simulink library "powerlib_models"  (Simulink 6.0)
settings: Solver=ode45  SolverMode=SingleTasking  StartTime=0.0  StopTime=10.0  RelTol=1e-3
values from neighbouring files (symbols this model uses):
  Ts = get(handles.edit1,'string')    [powergui.m]
undefined symbols (not defined in the file or in its folder): A, a0, a1, a2, a3, a4, a5, Ac, Amplitude, Amplitudes, B, BaseCurrent, BaseFlux, Bc, C, Capacitance, Cc, Columns, ConnectionType, Cs, ctrl, current, Current, damp, Dc, Dd, DiscIntNeverNeededParam, dref, dwo, exc, excAxis, F, Flux, fnom, Frequency, FreqVps, Gain1, gate, GH, GHd, GI, GId, GL, GLd, H, HarmonicGeneration, HT, hyd, I1_init, ib, ib2, Id1o, Inductance, InitialFlux, InitialSlope, io, Iq1o, isfinite, j, J ... (+138)
libraries: powerlib_models x32, powerlib_extras x4
(part 5 of 11)

== system powerlib_models/Phasors/SM_mechanics ==
  note: This subsystem models the mechanical part of the machine.
  Te : Inport  Port=1  PortDimensions=1  LatchInput=off
  Pm : Inport  Port=2  LatchInput=off
  1_(2H) : Gain  Gain=1/(2*H)  SaturateOnIntegerOverflow=on
  1_Pb : Gain  Gain=1/Pb  SaturateOnIntegerOverflow=on
  Clock : Clock
      settings: Decimation=10
  F1 : Gain  Orientation=left  Gain=F  SaturateOnIntegerOverflow=on
  Integrator : Integrator  InitialCondition=dwo
  Integrator1 : Integrator  InitialCondition=tho
  Integrator2 : Integrator  InitialCondition=tho
  Mux1 : Mux  Inputs=2
  Mux2 : Mux  Inputs=6
  Product : Product  SaturateOnIntegerOverflow=on  InputSameDT=on
  Sum : Sum  SaturateOnIntegerOverflow=on  InputSameDT=on
  Sum2 : Sum  Inputs=+--  SaturateOnIntegerOverflow=on  InputSameDT=on
  Sum3 : Sum  SaturateOnIntegerOverflow=on  InputSameDT=on
  div : Fcn  Expr=u[2]/u[1]
      mask Display: disp('/')
  nom. speed : Constant
  theta : Gain  Gain=180/pi  SaturateOnIntegerOverflow=on
  units : Gain  Gain=Nb  SaturateOnIntegerOverflow=on
  units1 : Gain  Gain=Pb  SaturateOnIntegerOverflow=on
  units2 : Gain  Gain=Pb/Nb  SaturateOnIntegerOverflow=on
  web1 : Gain  Gain=web_psb  SaturateOnIntegerOverflow=on
  web2 : Gain  Gain=web_psb  SaturateOnIntegerOverflow=on
  web3 : Gain  Gain=web_psb  SaturateOnIntegerOverflow=on
  misc : Outport  InitialOutput=0
  thetae : Outport  Port=2  InitialOutput=0
  we : Outport  Port=3  InitialOutput=0
  wires:
  Sum3/1 -> thetae/1
  Mux2/1 -> misc/1
  Sum/1 -> F1/1, Product/1, web3/1, units/1, Mux1/1, we/1  "n"
  Sum2/1 -> 1_(2H)/1
  F1/1 -> Sum2/3
  1_Pb/1 -> Mux1/2
  Pm/1 -> 1_Pb/1
  Mux1/1 -> div/1
  Te/1 -> Product/2, Sum2/2, units2/1  "Te"
  div/1 -> Sum2/1
  1_(2H)/1 -> Integrator/1
  nom. speed/1 -> Sum/1
  Product/1 -> units1/1  "Pe"
  Integrator/1 -> Sum/2, web1/1, Mux2/4  "dw"
  web1/1 -> Integrator2/1
  Clock/1 -> web2/1
  web2/1 -> Sum3/2
  Integrator2/1 -> Sum3/1, Mux2/1  "d_theta (rad)"
  Integrator1/1 -> theta/1  "d_theta (rad)"
  web3/1 -> Integrator1/1
  theta/1 -> Mux2/5  "theta"
  units/1 -> Mux2/2
  units1/1 -> Mux2/3
  units2/1 -> Mux2/6

== system powerlib_models/Phasors/SSM_mechanics ==
  Pm : Inport  Port=1  LatchInput=off
  Pe : Inport  Port=2  LatchInput=off
  1_(2*H) : Gain  Gain=1/(2*H)  SaturateOnIntegerOverflow=on
  1_Pb : Gain  Gain=1/Pb  SaturateOnIntegerOverflow=on
  Gain : Gain  Orientation=left  Gain=Kd  SaturateOnIntegerOverflow=on
  Integrator : Integrator  InitialCondition=dwo
  Integrator1 : Integrator  InitialCondition=tho
  Mux1 : Mux  Inputs=2
  Sum : Sum  SaturateOnIntegerOverflow=on  InputSameDT=on
  Sum1 : Sum  Inputs=+-  SaturateOnIntegerOverflow=on  InputSameDT=on
  Sum2 : Sum  Inputs=-+  SaturateOnIntegerOverflow=on  InputSameDT=on
  div : Fcn  Expr=u[2]/u[1]
      mask Display: disp('division')
  nom. speed : Constant
  web : Gain  Gain=web  SaturateOnIntegerOverflow=on
  theta_e : Outport  InitialOutput=0
  wm : Outport  Port=2  InitialOutput=0
  wires:
  nom. speed/1 -> Sum/1
  Integrator/1 -> Gain/1, Sum/2
  Sum1/1 -> 1_(2*H)/1
  Gain/1 -> Sum1/2
  div/1 -> Sum1/1
  1_(2*H)/1 -> Integrator/1
  Sum/1 -> web/1, wm/1, Mux1/1
  Sum2/1 -> Mux1/2
  Pe/1 -> Sum2/1
  Mux1/1 -> div/1
  Integrator1/1 -> theta_e/1
  web/1 -> Integrator1/1
  1_Pb/1 -> Sum2/2
  Pm/1 -> 1_Pb/1

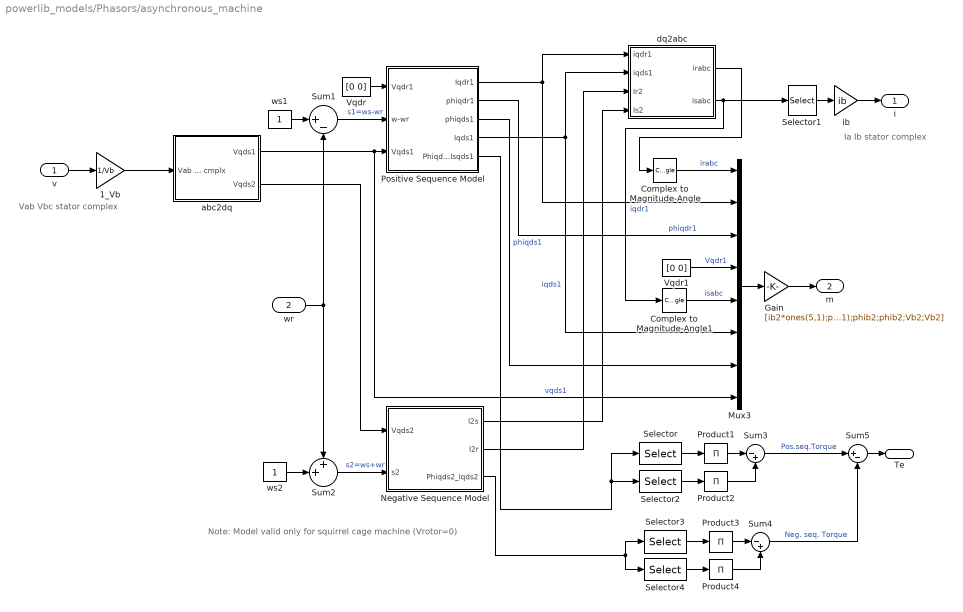
== system powerlib_models/Phasors/asynchronous_machine ==
  note: Note: Model valid only for squirrel cage machine (Vrotor=0)
  note: Ia Ib stator
      | complex
  note: Vab Vbc stator
      | complex
  v : Inport  Port=1  LatchInput=off
  wr : Inport  Port=2  LatchInput=off
  1_Vb : Gain  Gain=1/Vb  SaturateOnIntegerOverflow=on
  Complex to Magnitude-Angle : ComplexToMagnitudeAngle  Output=Magnitude
  Complex to Magnitude-Angle1 : ComplexToMagnitudeAngle  Output=Magnitude
  Gain : Gain  Gain=[ib2*ones(5,1);phib2;phib2;Vb2;Vb2;ib2*ones(5,1);phib2;phib2;Vb2;Vb2]  SaturateOnIntegerOverflow=on
  Mux3 : Mux  Inputs=[3,2,2,2,3,2,2,2]
  Negative Sequence Model : Subsystem
  Positive Sequence Model : Subsystem
  Product{1..4} (4 alike) : Product  Inputs=1  SaturateOnIntegerOverflow=on  InputSameDT=on
  Selector : Selector  Elements=[1 4]  InputPortWidth=4
  Selector1 : Selector  Elements=[1 2]  InputPortWidth=3
  Selector2 : Selector  Elements=[2 3]  InputPortWidth=4
  Selector3 : Selector  Elements=[1 4]  InputPortWidth=4
  Selector4 : Selector  Elements=[2 3]  InputPortWidth=4
  Sum1 : Sum  Inputs=|+-  SaturateOnIntegerOverflow=on  InputSameDT=on
  Sum2 : Sum  Inputs=++|  SaturateOnIntegerOverflow=on  InputSameDT=on
  Sum3 : Sum  Inputs=|-+  SaturateOnIntegerOverflow=on  InputSameDT=on
  Sum4 : Sum  Inputs=|-+  SaturateOnIntegerOverflow=on  InputSameDT=on
  Sum5 : Sum  Inputs=|+-  SaturateOnIntegerOverflow=on  InputSameDT=on
  Vqdr : Constant  Value=[0 0]
  Vqdr1 : Constant  Value=[0 0]
  abc2dq : Subsystem
  dq2abc : Subsystem
  ib : Gain  Gain=ib  SaturateOnIntegerOverflow=on
  ws1 : Constant
  ws2 : Constant
  i : Outport
  m : Outport  Port=2
  Te : Outport  Port=3
  wires:
  Negative Sequence Model/2(I2r) -> dq2abc/3(Ir2)
  Negative Sequence Model/1(I2s) -> dq2abc/4(Is2)
  Positive Sequence Model/3(phiqds1) -> Mux3/7  "phiqds1"
  Positive Sequence Model/2(phiqdr1) -> Mux3/3  "phiqdr1"
  abc2dq/2(Vqds2) -> Negative Sequence Model/1(Vqds2)
  Sum2/1 -> Negative Sequence Model/2(s2)  "s2=ws+wr"
  ib/1 -> i/1
  Mux3/1 -> Gain/1
  Gain/1 -> m/1
  dq2abc/2(isabc) -> Complex to Magnitude-Angle1/1, Selector1/1
  dq2abc/1(irabc) -> Complex to Magnitude-Angle/1
  Positive Sequence Model/1(Iqdr1) -> Mux3/2, dq2abc/1(iqdr1)  "iqdr1"
  abc2dq/1(Vqds1) -> Positive Sequence Model/3(Vqds1), Mux3/8  "vqds1"
  Positive Sequence Model/4(Iqds1) -> dq2abc/2(iqds1), Mux3/6  "iqds1"
  Vqdr/1 -> Positive Sequence Model/1(Vqdr1)
  1_Vb/1 -> abc2dq/1(Vab Vbc cmplx)
  v/1 -> 1_Vb/1
  Selector1/1 -> ib/1
  Complex to Magnitude-Angle/1 -> Mux3/1  "irabc"
  Complex to Magnitude-Angle1/1 -> Mux3/5  "isabc"
  ws1/1 -> Sum1/1
  Sum1/1 -> Positive Sequence Model/2(w-wr)  "s1=ws-wr"
  Vqdr1/1 -> Mux3/4  "Vqdr1"
  ws2/1 -> Sum2/2
  wr/1 -> Sum2/1, Sum1/2
  Positive Sequence Model/5(Phiqds1_Isqds1) -> Selector2/1, Selector/1
  Negative Sequence Model/3(Phiqds2_Iqds2) -> Selector3/1, Selector4/1
  Sum4/1 -> Sum5/2  "Neg. seq. Torque"
  Sum3/1 -> Sum5/1  "Pos.seq.Torque"
  Product3/1 -> Sum4/1
  Product4/1 -> Sum4/2
  Selector4/1 -> Product4/1
  Selector3/1 -> Product3/1
  Product1/1 -> Sum3/1
  Product2/1 -> Sum3/2
  Selector2/1 -> Product2/1
  Selector/1 -> Product1/1
  Sum5/1 -> Te/1

== system powerlib_models/Phasors/breaker ==
  "v " : Inport  Port=1  LatchInput=off
  g : Inport  Port=2  LatchInput=off
  Constant : Constant  Value=complex(zeros(Nsw,1),zeros(Nsw,1))
  Terminator : Terminator
  i : Outport  InitialOutput=0
  Status : Outport  Port=2  InitialOutput=0
  wires:
  Constant/1 -> i/1
  g/1 -> Status/1
  "v "/1 -> Terminator/1  "Vak"

== system powerlib_models/Phasors/distributed_param_line ==
  v : Inport  Port=1  LatchInput=off
  Constant : Constant  Value=complex(zeros(1,2*nphase),zeros(1,2*nphase))
  Terminator : Terminator
  i : Outport  InitialOutput=0
  wires:
  v/1 -> Terminator/1
  Constant/1 -> i/1

== system powerlib_models/Phasors/ideal_switch ==
  v : Inport  Port=1  LatchInput=off
  g : Inport  Port=2  LatchInput=off
  1/Rsw : Gain  Gain=1./Rsw  SaturateOnIntegerOverflow=on
  1/Rsw1 : Gain  Gain=0  SaturateOnIntegerOverflow=on
  Constant : Constant  Value=complex(zeros(Nsw,1),zeros(Nsw,1))
  Mux : Mux  Inputs=2
  Switch : Switch  Threshold=0.5  InputSameDT=on
  i : Outport  InitialOutput=0
  Status : Outport  Port=2  InitialOutput=0
  m : Outport  Port=3  InitialOutput=0
  wires:
  1/Rsw1/1 -> Switch/3
  Switch/1 -> Mux/1
  1/Rsw/1 -> Switch/1  "Iak"
  v/1 -> Mux/2, 1/Rsw/1, 1/Rsw1/1  "Vak"
  Mux/1 -> m/1  "measurement signals"
  g/1 -> Status/1, Switch/2
  Constant/1 -> i/1

== system powerlib_models/Phasors/simplified_sync_mach ==
  note: ia ib complex
  note: Vab Vbc
      | complex
  v : Inport  Port=1  LatchInput=off
  e : Inport  Port=2  LatchInput=off
  theta_e : Inport  Orientation=left  Port=3  LatchInput=off
  wm : Inport  Port=4  LatchInput=off
  1_Vb : Gain  Gain=1/Vb  SaturateOnIntegerOverflow=on
  Complex to Magnitude-Angle : ComplexToMagnitudeAngle  Output=Magnitude
  Complex to Magnitude-Angle1 : ComplexToMagnitudeAngle  Output=Magnitude
  Constant4 : Constant  Orientation=left  Value=web
  Filter_T=1ms : StateSpace  A=-1e3*eye(3)  B=1e3*eye(3)  C=eye(3)  D=zeros(3)
  "Idq1 Idq2 Pe " : Subsystem
  Integrator : Integrator  Orientation=left
  LL2LN : Subsystem
  Mux1 : Mux  Inputs=3
  Phasors Ia Ib : Subsystem
  Subsystem : Subsystem
  Sum6 : Sum  Orientation=left  Inputs=+-  SaturateOnIntegerOverflow=on  InputSameDT=on
  ib1 : Gain  Gain=ib  SaturateOnIntegerOverflow=on
  i : Outport  InitialOutput=0
  m : Outport  Port=2  InitialOutput=0
  Pe : Outport  Port=3  InitialOutput=0
  wires:
  Mux1/1 -> Subsystem/3(e)
  Complex to Magnitude-Angle1/1 -> Filter_T=1ms/1
  LL2LN/1(Vabc_n) -> Complex to Magnitude-Angle1/1  "Line-to-neutral voltages"
  Complex to Magnitude-Angle/1 -> Subsystem/1(i)
  Phasors Ia Ib/1(Iabc cmplx) -> Complex to Magnitude-Angle/1
  "Idq1 Idq2 Pe "/1(Pe) -> Subsystem/6(Pe), Pe/1  "Pe"
  Sum6/1 -> Subsystem/4(theta), "Idq1 Idq2 Pe "/3(delta)  "theta"
  Integrator/1 -> Sum6/2
  Constant4/1 -> Integrator/1
  ib1/1 -> i/1
  Phasors Ia Ib/2(Iab cmplx) -> ib1/1
  e/1 -> Mux1/3, Mux1/1, Mux1/2, "Idq1 Idq2 Pe "/2(e)  "Internal volltage  magnitudes"
  1_Vb/1 -> LL2LN/1(Vab_bc), "Idq1 Idq2 Pe "/1(Vab Vbc cmplx)
  v/1 -> 1_Vb/1
  Subsystem/1(*) -> m/1
  "Idq1 Idq2 Pe "/2(Idq1) -> Phasors Ia Ib/1(Idq1)
  "Idq1 Idq2 Pe "/3(Idq2) -> Phasors Ia Ib/2(Idq2)
  Filter_T=1ms/1 -> Subsystem/2(v)
  theta_e/1 -> Sum6/1
  wm/1 -> Subsystem/5(wm)

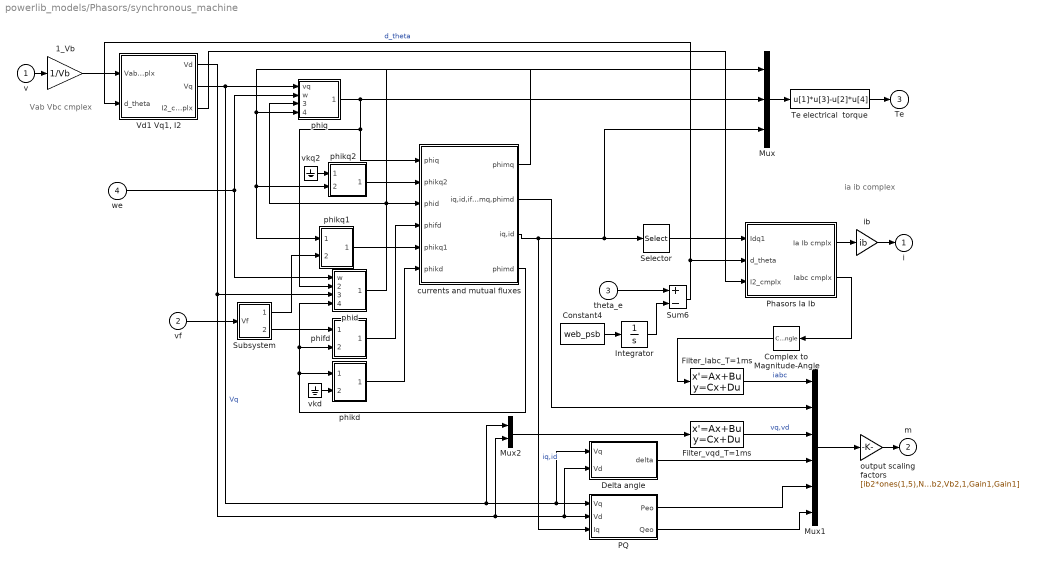
== system powerlib_models/Phasors/synchronous_machine ==
  note: Vab Vbc cmplex
  note: ia ib complex
  v : Inport  Port=1  LatchInput=off
  vf : Inport  Port=2  LatchInput=off
  theta_e : Inport  Port=3  LatchInput=off
  we : Inport  Port=4  LatchInput=off
  1_Vb : Gain  Gain=1/Vb  SaturateOnIntegerOverflow=on
  Complex to Magnitude-Angle : ComplexToMagnitudeAngle  Orientation=left  Output=Magnitude
  Constant4 : Constant  Value=web_psb
  Delta angle : Subsystem
  Filter_Iabc_T=1ms : StateSpace  A=-1e3*eye(3)  B=1e3*eye(3)  C=eye(3)  D=zeros(3)
  Filter_vqd_T=1ms : StateSpace  A=-1e3*eye(2)  B=1e3*eye(2)  C=eye(2)  D=zeros(2)  X0=[phido -phiqo]
  Integrator : Integrator
  Mux : Mux  Inputs=[ 1 1 2 ]
  Mux1 : Mux  Inputs="[ 3 8 2  1 1 1]"
  Mux2 : Mux  Inputs=2
  PQ : Subsystem
  Phasors Ia Ib : Subsystem
  Selector : Selector  Elements=[2 1]  InputPortWidth=2
  Subsystem : Subsystem
  Sum6 : Sum  Inputs=+-  SaturateOnIntegerOverflow=on  InputSameDT=on
  Te electrical  torque : Fcn  Expr=u[1]*u[3]-u[2]*u[4]
  "Vd1 Vq1, I2 " : Subsystem
  currents and mutual fluxes : Subsystem
  ib : Gain  Gain=ib  SaturateOnIntegerOverflow=on
  output scaling factors : Gain  Gain=[ib2*ones(1,5),N2,ib2,ib2,ib2,phib,phib,Vb2,Vb2,1,Gain1,Gain1]
  phid : Subsystem
      mask Display: disp('phid')
  phifd : Subsystem
      mask Display: disp('phifd')
  phikd : Subsystem
      mask Display: disp('phikd')
  phikq1 : Subsystem
      mask Display: disp('phikq1')
  phikq2 : Subsystem
      mask Display: disp('phikq2')
  phiq : Subsystem
      mask Display: disp('phiq')
  vkd : Ground
  vkq2 : Ground
  i : Outport  InitialOutput=0
  m : Outport  Port=2  InitialOutput=0
  Te : Outport  Port=3  InitialOutput=0
  wires:
  PQ/2(Qeo) -> Mux1/6
  PQ/1(Peo) -> Mux1/5
  Delta angle/1(delta) -> Mux1/4
  Complex to Magnitude-Angle/1 -> Filter_Iabc_T=1ms/1
  Phasors Ia Ib/2(Iabc cmplx) -> Complex to Magnitude-Angle/1
  ib/1 -> i/1
  Phasors Ia Ib/1(Ia Ib cmplx) -> ib/1
  currents and mutual fluxes/1(phimq) -> phiq/4(phimq), phikq1/1(phimq), phikq2/2(phimq)
  currents and mutual fluxes/4(phimd) -> phid/4(phimd), phifd/2(phimd), phikd/1(phimd)
  phiq/1(phiq) -> currents and mutual fluxes/1(phiq), phid/2(phiq), Mux/2
  "Vd1 Vq1, I2 "/1(Vd) -> phid/3(vd), PQ/2(Vd), Delta angle/2(Vd), Mux2/2
  "Vd1 Vq1, I2 "/2(Vq) -> phiq/1(vq), PQ/1(Vq), Delta angle/1(Vq), Mux2/1  "Vq"
  phid/1(phid) -> phiq/3(phid), currents and mutual fluxes/3(phid), Mux/1
  Selector/1 -> Phasors Ia Ib/1(Idq1)
  Mux2/1 -> Filter_vqd_T=1ms/1
  "Vd1 Vq1, I2 "/3(I2_cmplx) -> Phasors Ia Ib/3(I2_cmplx)
  Integrator/1 -> Sum6/2
  Constant4/1 -> Integrator/1
  Sum6/1 -> Phasors Ia Ib/2(d_theta), "Vd1 Vq1, I2 "/2(d_theta)  "d_theta"
  phikq2/1(phikq2) -> currents and mutual fluxes/2(phikq2)
  phikq1/1(phikq1) -> currents and mutual fluxes/5(phikq1)
  phifd/1(phifd) -> currents and mutual fluxes/4(phifd)
  phikd/1(phikd) -> currents and mutual fluxes/6(phikd)
  output scaling factors/1 -> m/1
  Mux1/1 -> output scaling factors/1
  currents and mutual fluxes/3(iq,id) -> PQ/3(Iq), Selector/1, Mux/3  "iq,id"
  currents and mutual fluxes/2("iq,id,ifd, ikq1,ikq2,ikd, phimq,phimd") -> Mux1/2
  v/1 -> 1_Vb/1
  1_Vb/1 -> "Vd1 Vq1, I2 "/1(Vab Vbc cmplx)
  Subsystem/2(Vfd) -> phifd/1(vfd)
  Subsystem/1(Vkq1) -> phikq1/2(vkq1)
  vkd/1 -> phikd/2(vkd)
  vkq2/1 -> phikq2/1(vkq2)
  vf/1 -> Subsystem/1(Vf)
  Filter_Iabc_T=1ms/1 -> Mux1/1  "iabc"
  Filter_vqd_T=1ms/1 -> Mux1/3  "vq,vd"
  theta_e/1 -> Sum6/1
  we/1 -> phid/1(w), phiq/2(w)
  Mux/1 -> Te electrical  torque/1
  Te electrical  torque/1 -> Te/1

== system powerlib_models/Sources/ThreePhaseSource ==
  Mux : Mux  Inputs=3
  Sine Wave A : Sin  Amplitude=Amplitude  Frequency=2*pi*Frequency  Phase=Phase*pi/180  SampleTime=Ts
  Sine Wave B : Sin  Amplitude=Amplitude  Frequency=2*pi*Frequency  Phase=(Phase-120)*pi/180  SampleTime=Ts
  Sine Wave C : Sin  Amplitude=Amplitude  Frequency=2*pi*Frequency  Phase=(Phase+120)*pi/180  SampleTime=Ts
  Out1 : Outport
  wires:
  Sine Wave B/1 -> Mux/2
  Sine Wave A/1 -> Mux/1
  Sine Wave C/1 -> Mux/3
  Mux/1 -> Out1/1

== system powerlib_models/Sources/ThreePhaseSource_Cmplx ==
  Constant : Constant  Value=complex(Amplitude*cos(Phase*pi/180),Amplitude*sin(Phase*pi/180))
  Constant1 : Constant  Value=complex(Amplitude*cos((Phase-120)*pi/180),Amplitude*sin((Phase-120)*pi/180))
  Constant2 : Constant  Value=complex(Amplitude*cos((Phase+120)*pi/180),Amplitude*sin((Phase+120)*pi/180))
  Mux : Mux  Inputs=3
  Out1 : Outport
  wires:
  Constant1/1 -> Mux/2
  Constant/1 -> Mux/1
  Constant2/1 -> Mux/3
  Mux/1 -> Out1/1

== system powerlib_models/Switch Current Source/IGBT ==
  v : Inport  Port=1  LatchInput=off
  g : Inport  Port=2  LatchInput=off
  Conduction Logic : Subsystem
  IC : InitialCondition  Value=IC
  Integrator : Integrator  ExternalReset=rising  InitialConditionSource=external  ShowStatePort=on
  L_device : Gain  Gain=1./Lon  SaturateOnIntegerOverflow=on
  Mux : Mux  Inputs=2
  R_device : Gain  Orientation=left  Gain=Ron  SaturateOnIntegerOverflow=on
  Switch : Switch  Threshold=eps  InputSameDT=on
  Tail : Subsystem
  Vak-VT-RT*Iak2 : Sum  Inputs=-|+|-  SaturateOnIntegerOverflow=on  InputSameDT=on
  Vf : Constant  Orientation=up  Value=Vf
  Vf1 : Constant  Value=0*IC
  Vf2 : Constant  Value=0
  i : Outport  InitialOutput=0
  m : Outport  Port=2  InitialOutput=0
  wires:
  Conduction Logic/1(status) -> Tail/2(switch), Integrator/2, Switch/2
  Integrator/1 -> R_device/1, Tail/1(iak)  "IGBT current"
  IC/1 -> Integrator/3
  Integrator/State -> Conduction Logic/1(iak)  "IGBT current"
  g/1 -> Conduction Logic/3(g)  "gate signal"
  Vak-VT-RT*Iak2/1 -> L_device/1
  Tail/1(Iak) -> Mux/1, i/1  "current"
  Mux/1 -> m/1
  Vf/1 -> Vak-VT-RT*Iak2/3
  v/1 -> Vak-VT-RT*Iak2/2, Conduction Logic/2(Vak), Mux/2  "IGBT voltage"
  R_device/1 -> Vak-VT-RT*Iak2/1
  Vf1/1 -> IC/1
  Switch/1 -> Integrator/1
  L_device/1 -> Switch/1
  Vf2/1 -> Switch/3

== system powerlib_models/Switch Current Source/detailed_thyristor ==
  v : Inport  Port=1  LatchInput=off
  g : Inport  Port=2  LatchInput=off
  Conduction logic : Subsystem
  Mux : Mux  Inputs=2
  Switch-Ron-Lon : Subsystem
  i : Outport  InitialOutput=0
  m : Outport  Port=2  InitialOutput=0
  wires:
  Conduction logic/1(reset) -> Switch-Ron-Lon/2(Reset)
  Mux/1 -> m/1
  Switch-Ron-Lon/1("Iak  ") -> i/1, Mux/1, Conduction logic/1(Iak_meas.)
  v/1 -> Switch-Ron-Lon/1(Vak), Conduction logic/2(Vak), Mux/2
  g/1 -> Conduction logic/3(G)

== system powerlib_models/Switch Current Source/diode ==
  v : Inport  Port=1  LatchInput=off
  0  1 : Constant  Value=0
  Conduction logic : Subsystem
  IC : InitialCondition  Value=IC
  Integrator1 : Integrator  ExternalReset=rising  InitialConditionSource=external  LimitOutput=on  LowerSaturationLimit=0
  Lon : Gain  Gain=1./Lon  SaturateOnIntegerOverflow=on
  Mux : Mux  Inputs=2
  Ron : Gain  Orientation=left  Gain=Ron  SaturateOnIntegerOverflow=on
  Test : Switch  Threshold=0.5  InputSameDT=on
  Vak-VT-RT*Iak2 : Sum  Inputs=-|+|-  SaturateOnIntegerOverflow=on  InputSameDT=on
  Vf : Constant  Orientation=up  Value=Vf
  Vf1 : Constant  Value=0*IC
  i : Outport  InitialOutput=0
  m : Outport  Port=2  InitialOutput=0
  wires:
  Mux/1 -> m/1
  v/1 -> Mux/2, Conduction logic/2(Vak), Vak-VT-RT*Iak2/2  "Diode voltage"
  IC/1 -> Integrator1/3
  Lon/1 -> Integrator1/1
  Conduction logic/1(status) -> Integrator1/2, Test/2
  Vak-VT-RT*Iak2/1 -> Lon/1
  Integrator1/1 -> Ron/1, Test/1  "Inductor current"
  Ron/1 -> Vak-VT-RT*Iak2/1
  Vf/1 -> Vak-VT-RT*Iak2/3
  Vf1/1 -> IC/1
  0  1/1 -> Test/3  "zero current"
  Test/1 -> i/1, Mux/1, Conduction logic/1(Iak)  "Diode current"

== system powerlib_models/Switch Current Source/gto ==
  v : Inport  Port=1  LatchInput=off
  g : Inport  Port=2  LatchInput=off
  Conduction Logic : Subsystem
  IC : InitialCondition  Value=IC
  Integrator : Integrator  ExternalReset=rising  InitialConditionSource=external  ShowStatePort=on
  L_device : Gain  Gain=1./Lon  SaturateOnIntegerOverflow=on
  Mux : Mux  Inputs=2
  R_device : Gain  Orientation=left  Gain=Ron  SaturateOnIntegerOverflow=on
  Switch : Switch  Threshold=eps  InputSameDT=on
  Tail : Subsystem
  Vak-VT-RT*Iak2 : Sum  Inputs=-|+|-  SaturateOnIntegerOverflow=on  InputSameDT=on
  Vf : Constant  Orientation=up  Value=Vf
  Vf1 : Constant  Value=0*IC
  Vf2 : Constant  Value=0
  i : Outport  InitialOutput=0
  m : Outport  Port=2  InitialOutput=0
  wires:
  Conduction Logic/1(status) -> Tail/2(switch), Integrator/2, Switch/2  "switch status"
  Integrator/1 -> Tail/1(iak), R_device/1  "GTO current"
  Integrator/State -> Conduction Logic/1(iak)  "GTO current"
  g/1 -> Conduction Logic/3(g)  "gate signal"
  R_device/1 -> Vak-VT-RT*Iak2/1
  Tail/1(Iak) -> i/1, Mux/1  "GTO current"
  Mux/1 -> m/1
  v/1 -> Vak-VT-RT*Iak2/2, Mux/2, Conduction Logic/2(Vak)  "GTO voltage"
  Vf/1 -> Vak-VT-RT*Iak2/3
  Vak-VT-RT*Iak2/1 -> L_device/1
  Vf1/1 -> IC/1
  IC/1 -> Integrator/3
  Switch/1 -> Integrator/1
  L_device/1 -> Switch/1
  Vf2/1 -> Switch/3

== system powerlib_models/Switch Current Source/mosfet ==
  v : Inport  Port=1  LatchInput=off
  g : Inport  Port=2  LatchInput=off
  0  1 : Constant  Value=0
  Conduction Logic : Subsystem
  IC : InitialCondition  Value=IC
  Integrator1 : Integrator  ExternalReset=rising  InitialConditionSource=external  LowerSaturationLimit=0  ShowStatePort=on
  Lon : Gain  Gain=1./Lon  SaturateOnIntegerOverflow=on
  Mux : Mux  Inputs=2
  R_device : Gain  Orientation=left  Gain=Ron  SaturateOnIntegerOverflow=on
  R_device1 : Gain  Orientation=left  Gain=Rd  SaturateOnIntegerOverflow=on
  Sign : Signum  Orientation=left
  Test : Switch  Threshold=0.5  InputSameDT=on
  Test4 : Switch  Orientation=left  Threshold=eps  InputSameDT=on
  Vds-Ron*Ids : Sum  Inputs=-+|  SaturateOnIntegerOverflow=on  InputSameDT=on
  Vf1 : Constant  Value=0*IC
  i : Outport  InitialOutput=0
  m : Outport  Port=2  InitialOutput=0
  wires:
  Integrator1/1 -> Test/1, Sign/1, R_device/1, R_device1/1  "mosfet current"
  Test/1 -> Mux/1, i/1
  Conduction Logic/1(status) -> Integrator1/2, Test/2
  Integrator1/State -> Conduction Logic/1(Ids_meas)  "mosfet current"
  v/1 -> Mux/2, Conduction Logic/2(Vds), Vds-Ron*Ids/2  "mosfet voltage"
  Sign/1 -> Test4/2
  R_device1/1 -> Test4/3
  Lon/1 -> Integrator1/1
  Vds-Ron*Ids/1 -> Lon/1
  R_device/1 -> Test4/1
  g/1 -> Conduction Logic/3(G)  "gate signal"
  Mux/1 -> m/1
  Test4/1 -> Vds-Ron*Ids/1
  0  1/1 -> Test/3  "zero current"
  Vf1/1 -> IC/1
  IC/1 -> Integrator1/3

== system powerlib_models/Switch Current Source/thyristor ==
  v : Inport  Port=1  LatchInput=off
  g : Inport  Port=2  LatchInput=off
  0  1 : Constant  Value=0
  Conduction Logic : Subsystem
  IC : InitialCondition  Value=IC
  Integrator : Integrator  ExternalReset=rising  InitialConditionSource=external  LimitOutput=on  LowerSaturationLimit=0
  Lon : Gain  Gain=1./Lon  SaturateOnIntegerOverflow=on
  Mux : Mux  Inputs=2
  R_device : Gain  Orientation=left  Gain=Ron  SaturateOnIntegerOverflow=on
  Test : Switch  Threshold=0.5  InputSameDT=on
  Vak-VT-RT*Iak2 : Sum  Inputs=-|+|-  SaturateOnIntegerOverflow=on  InputSameDT=on
  Vf : Constant  Orientation=up  Value=Vf
  Vf1 : Constant  Value=0*IC
  i : Outport  InitialOutput=0
  m : Outport  Port=2  InitialOutput=0
  wires:
  g/1 -> Conduction Logic/3("G ")  "gate signal"
  Conduction Logic/1(Status) -> Integrator/2, Test/2
  Mux/1 -> m/1
  Lon/1 -> Integrator/1
  Integrator/1 -> R_device/1, Test/1  "Inductor current"
  v/1 -> Conduction Logic/2(Vak), Mux/2, Vak-VT-RT*Iak2/2  "thyristor voltage"
  Vak-VT-RT*Iak2/1 -> Lon/1
  IC/1 -> Integrator/3
  R_device/1 -> Vak-VT-RT*Iak2/1
  Vf/1 -> Vak-VT-RT*Iak2/3
  Vf1/1 -> IC/1
  Test/1 -> i/1, Mux/1, Conduction Logic/1("Iak ")  "Thyiristor Current"
  0  1/1 -> Test/3  "zero current"

== system powerlib_models/Continuous/3_Phase_Prog_Source/Harmonic A generation ==
  Enable : Inport  Port=1  LatchInput=off
  Clock : Clock
  Gain2 : Gain  Gain=2*pi*n_Harmo  SaturateOnIntegerOverflow=on
  Gain3 : Gain  Gain=pi/180  SaturateOnIntegerOverflow=on
  Multiport Switch : MultiPortSwitch  Inputs=3  InputSameDT=on
  Negative-sequence : Constant  Value=[0 2*pi/3 -2*pi/3]
  Phase_Harmo : Constant  Value=Phase_Harmo
  Phase_Harmo1 : Constant  Value=Mag_Harmo
  Phase_Harmo2 : Constant  Value=Seq_Harmo
  Positive-sequence : Constant  Value=[0 -2*pi/3 2*pi/3]
  Product : Product  SaturateOnIntegerOverflow=on  InputSameDT=on
  Product1 : Product  Inputs=3  SaturateOnIntegerOverflow=on  InputSameDT=on
  Sum : Sum  Inputs=+++  SaturateOnIntegerOverflow=on  InputSameDT=on
  Sum1 : Sum  SaturateOnIntegerOverflow=on  InputSameDT=on
  Trigonometric Function1 : Trigonometry
  Zero-sequence : Constant  Value=[0 0 0]
  valp_nom1 : Constant  Value=Freq_Vps
  valp_nom2 : Constant
  HarmoA : Outport
  wires:
  Gain3/1 -> Sum/2
  Phase_Harmo/1 -> Gain3/1
  Enable/1 -> Product1/1
  valp_nom2/1 -> Sum1/2
  Phase_Harmo2/1 -> Sum1/1
  Sum1/1 -> Multiport Switch/1
  Phase_Harmo1/1 -> Product1/2
  Product1/1 -> HarmoA/1
  Trigonometric Function1/1 -> Product1/3
  Product/1 -> Sum/1
  Clock/1 -> Product/1
  Gain2/1 -> Product/2
  valp_nom1/1 -> Gain2/1
  Negative-sequence/1 -> Multiport Switch/4
  Positive-sequence/1 -> Multiport Switch/3
  Zero-sequence/1 -> Multiport Switch/2
  Multiport Switch/1 -> Sum/3
  Sum/1 -> Trigonometric Function1/1

== system powerlib_models/Continuous/3_Phase_Prog_Source/Harmonic B generation ==
  Enable : Inport  Port=1  LatchInput=off
  Clock1 : Clock
  Gain2 : Gain  Gain=2*pi*n_Harmo  SaturateOnIntegerOverflow=on
  Gain3 : Gain  Gain=pi/180  SaturateOnIntegerOverflow=on
  Multiport Switch : MultiPortSwitch  Inputs=3  InputSameDT=on
  Negative-sequence : Constant  Value=[0 2*pi/3 -2*pi/3]
  Phase_Harmo : Constant  Value=Phase_Harmo
  Phase_Harmo1 : Constant  Value=Mag_Harmo
  Phase_Harmo2 : Constant  Value=Seq_Harmo
  Positive-sequence : Constant  Value=[0 -2*pi/3 2*pi/3]
  Product : Product  SaturateOnIntegerOverflow=on  InputSameDT=on
  Product1 : Product  Inputs=3  SaturateOnIntegerOverflow=on  InputSameDT=on
  Sum : Sum  Inputs=+++  SaturateOnIntegerOverflow=on  InputSameDT=on
  Sum1 : Sum  SaturateOnIntegerOverflow=on  InputSameDT=on
  Trigonometric Function1 : Trigonometry
  Zero-sequence : Constant  Value=[0 0 0]
  valp_nom1 : Constant  Value=Freq_Vps
  valp_nom2 : Constant
  HarmoB : Outport
  wires:
  Gain3/1 -> Sum/2
  Phase_Harmo/1 -> Gain3/1
  Sum/1 -> Trigonometric Function1/1
  Multiport Switch/1 -> Sum/3
  Zero-sequence/1 -> Multiport Switch/2
  Positive-sequence/1 -> Multiport Switch/3
  Negative-sequence/1 -> Multiport Switch/4
  valp_nom1/1 -> Gain2/1
  Gain2/1 -> Product/2
  Clock1/1 -> Product/1
  Product/1 -> Sum/1
  Trigonometric Function1/1 -> Product1/3
  Product1/1 -> HarmoB/1
  Phase_Harmo1/1 -> Product1/2
  Sum1/1 -> Multiport Switch/1
  Phase_Harmo2/1 -> Sum1/1
  valp_nom2/1 -> Sum1/2
  Enable/1 -> Product1/1

== system powerlib_models/Continuous/3_Phase_Prog_Source/Timer ==
  Clock : Clock
  Look-Up Table : Lookup  DialogController=Simulink.DDGSource  InputValues=tv  OutputValues=opv  SaturateOnIntegerOverflow=on
  Out : Outport
  wires:
  Look-Up Table/1 -> Out/1
  Clock/1 -> Look-Up Table/1

== system powerlib_models/Continuous/3_Phase_Prog_Source/Variation SubSystem ==
  VariationType : Inport  Port=1  LatchInput=off
  Constant : Constant  Value=2
  Constant1 : Constant  Value=0
  Constant2 : Constant
  Constant3 : Constant
  Constant4 : Constant  Value=0
  Constant5 : Constant  Value=0
  Data Type  Conversion1 : DataTypeConversion  OutDataTypeMode=boolean  SaturateOnIntegerOverflow=on  RndMeth=Zero
  Data Type  Conversion2 : DataTypeConversion  Orientation=up  OutDataTypeMode=boolean  SaturateOnIntegerOverflow=on  RndMeth=Zero
  Gain1 : Gain  Gain=2*pi  SaturateOnIntegerOverflow=on
  Integrator : Integrator
  Logical Operator : Logic
  Logical Operator1 : Logic  Orientation=up  Operator=NOT
  Memory : Memory  Orientation=left
  Multiport Switch1 : MultiPortSwitch  InputSameDT=on
  Product : Product  SaturateOnIntegerOverflow=on  InputSameDT=on
  Product1 : Product  SaturateOnIntegerOverflow=on  InputSameDT=on
  Product2 : Product  SaturateOnIntegerOverflow=on  InputSameDT=on
  Relational Operator : RelationalOperator  Operator===  InputSameDT=on
  Relational Operator1 : RelationalOperator  Operator===  InputSameDT=on
  Step : Step  Time=Ton_Variation  SampleTime=0
  Step1 : Step  Time=Toff_Variation  Before=1  After=0  SampleTime=0
  Switch{,1..3} (4 alike) : Switch  Threshold=0.5  InputSameDT=on
  Trigonometric Function1 : Trigonometry
  valp_nom6 : Constant  Value=VariationStep
  valp_nom7 : Constant  Value=VariationRate
  valp_nom8 : Constant  Value=VariationMag
  valp_nom9 : Constant  Value=VariationFreq
  Value : Outport
  wires:
  Data Type  Conversion1/1 -> Logical Operator/2
  Constant5/1 -> Multiport Switch1/5
  Logical Operator1/1 -> Logical Operator/1
  Logical Operator/1 -> Switch3/2
  Step1/1 -> Switch2/2, Data Type  Conversion2/1  "Toff"
  Constant3/1 -> Relational Operator1/2
  Switch3/1 -> Value/1
  Switch2/1 -> Switch3/3, Memory/1
  Constant1/1 -> Switch3/1
  Memory/1 -> Switch2/3
  Multiport Switch1/1 -> Switch2/1
  Step/1 -> Product2/2, Switch/2  "Ton"
  VariationType/1 -> Relational Operator/1, Relational Operator1/1, Multiport Switch1/1
  Integrator/1 -> Multiport Switch1/3, Product1/1  "Ramp"
  Product2/1 -> Multiport Switch1/2  "Step"
  valp_nom6/1 -> Product2/1
  Relational Operator/1 -> Switch1/2
  Switch/1 -> Integrator/1
  Constant/1 -> Relational Operator/2
  Switch1/1 -> Switch/1
  Constant4/1 -> Switch/3
  Constant2/1 -> Switch1/3
  valp_nom7/1 -> Switch1/1
  Product/1 -> Multiport Switch1/4  "Mod"
  Product1/1 -> Trigonometric Function1/1
  Gain1/1 -> Product1/2
  valp_nom9/1 -> Gain1/1
  valp_nom8/1 -> Product/1
  Trigonometric Function1/1 -> Product/2
  Data Type  Conversion2/1 -> Logical Operator1/1
  Relational Operator1/1 -> Data Type  Conversion1/1

== system powerlib_models/Continuous/Dynamic_Load/3-phase PLL1 ==
  note: 3-phase PLL
  note: Pierre Giroux, Gilbert Sybille
      | Power System Laboratory, IREQ
      | Hydro-Quebec
  Vab_bc (pu) : Inport  Port=1  PortDimensions=2  LatchInput=off
  2nd-Order Filter : Subsystem  AncestorBlock=|  mask(2nd-Order Filter){FilterType=Lowpass, Fo=25, Zeta=0.707, Initialize=on, Vac_Init=[0 0 60], Vdc_Init=Finit, PlotResponse=off, param1=[1 1000 0.5]}
      | powerlib_extras/Control 
      | Blocks/2nd-Order
      | Filter
      mask prompts: FilterType "Filter Type:"; Fo "Cut-off frequency (Hz):"; Zeta "Damping factor Zeta ( Q = 1 / (2*Zeta) ):"; Initialize "Initialize filter states"; Vac_Init "AC initial input: [ Mag  Phase(degrees)  Freq(Hz) ]"; Vdc_Init "DC Initial input:"; PlotResponse "Plot filter response"; param1 "Frequency range(Hz) : [Start  End  Inc.]"
      mask init:
      | Wo=2*pi*Fo;
      | str=sprintf(' Fo=%iHz\n\n',Fo);
      | switch FilterType
      | case 1, % Lowpass
      |        X=[0 1 2 3 4];
      |        Y=[-2 -2 -3 -4 -4];
      |        n2=0;n1=0;n0=Wo*Wo;
      |        d2=1;d1=2*Zeta*Wo;d0=Wo*Wo;
      |  case 2,   % Highpass
      |        X=[0 1 2 3 4];
      |        Y=[-4 -4 -3 -2 -2];
      |        n2=1;n1=0;n0=0;
      |        d2=1;d1=2*Zeta*Wo;d0=Wo*Wo;
      |     case 3,   % Bandpass
      |        X=[0 1 2 3 4 5 ];
      |        Y=[-3 -3 -2 -2 -3 -3];
      |        n2=0;n1=2*Zeta*Wo;n0=0;
      |        d2=1;d1=2*Zeta*Wo;d0=Wo*Wo;
      |     case 4,  %Bandstop (Notch)
      |        X=[0 1 2 3 4 5 ];
      |        Y=[-2 -2 -3 -3 -2 -2];
      |        n2=1;n1=0;n0=Wo*Wo;
      |        d2=1;d1=2*Zeta*Wo;d0=Wo*Wo;
      |     end
      | %
      | numc=[n2 n1 n0];
      | denc=[d2 d1 d0];
      | [Ac,Bc,Cc,Dc]=tf2ss(numc,denc);
      | %
      | if Initialize==1  % Compute initial conditions on states
      | u1=Vac_Init(1)*exp(j*Vac_Init(2)*pi/180);
      | u2=Vdc_Init*exp(j*90*pi/180);
      | u=u1+u2;
      | u0=imag(u); % input at  t=0;
      | I=eye(size(Ac));
      | sI1=I*j*(2*pi*Vac_Init(3));
      | sI2=I*j*0;
      | x=inv(sI1-Ac)*Bc*u1 + inv(sI2-Ac)*Bc*u2;
      | x0c=imag(x);
      | else
      | x0c=0;
      | end
      | %
      | if PlotResponse==1 % Plot frequency and step response
      | figure(1)
      | sys=ss(Ac,Bc,Cc,Dc);
      | f=param1(1):param1(3):param1(2);
      | w=2*pi*f;
      | [mag phase]=bode(sys,w);
      | subplot(2,1,1)
      | plot(f,squeeze(mag))
      | title('Magnitude')
      | grid
      | subplot(2,1,2)
      | plot(f,squeeze(phase))
      | title('Phase (degrees)')
      | xlabel('Hz')
      | grid
      | figure(2)
      | step(sys)
      | end
      mask StyleString: popup(Lowpass|Highpass|Bandpass|Bandstop (Notch)),edit,edit,checkbox,edit,edit,checkbox,edit
      mask CallbackString: |||parametres=get_param(gcb,'MaskValues');p4=parametres{4};p7=parametres{7};if strcmp(p4,'on');param5='on';param6='on';else;param5='off';param6='off';end;if strcmp(p7,'on');param8='on';else;param8='off';end;visible={'on','on','on','on',param5,param6,'on',param8};set_param(gcb,'MaskVisibilities',visible)|||parametres=get_param(gcb,'MaskValues');p4=parametres{4};p7=parametres{7};if strcmp(p4,'on');param5='on';param6='on';else;param5='off';param6='off';end;if strcmp(p7,'on');param8='on';else;param8='off';end;visible={'on','on','on','on',param5,param6,'on',param8};set_param(gcb,'MaskVisibilities',visible)|
      mask Display:
      | plot(X,Y);
      | disp(str);
  Constant4 : Constant  Value=2*pi
  Discrete PI Controller : Subsystem  mask(Discrete PI Controller){Kp=Kp, Ki=Ki, Par_Limits=2*pi*Finit*[1.25 0.75], Init=2*pi*Finit}
      mask prompts: Kp "Proportional gain (Kp):"; Ki "Integral gain (Ki):"; Par_Limits "Output limits: [ Upper   Lower ]"; Init "Output initial value:"
      mask help: This block implements a discrete PI controller.
      mask init:
      | UpperLimit=Par_Limits(1);
      | LowerLimit=Par_Limits(2);
      mask Display: disp('PI');
  Gain10 : Gain  Gain=1/2/pi  SaturateOnIntegerOverflow=on
  Integrator : Integrator  InitialCondition=Phase_Init*pi/180  LimitOutput=on
  Math Function : Math  Operator=mod  SaturateOnIntegerOverflow=on
  Mux2 : Mux  Inputs=2
  Rate Limiter : RateLimiter  RisingSlewLimit=12  FallingSlewLimit=-12
  Trigonometric Function : Trigonometry
  Trigonometric Function2 : Trigonometry  Operator=cos
  Variable Frequency Mean value : Subsystem  mask(Variable-Frequency Mean Value){Finit=Finit, Vinit=0}
      mask prompts: Finit "Initial frequency (Hz):"; Vinit "Initial input (DC component):"
      mask help:
      | This  block computes the mean value of the input signal (port In) over a running window of one cycle of a specified frequency (port Freq).
      |
      | For the first cycle of simulation (specified by the parameter "Initial frequency"), the ouput is held to the value of the  "Initial input" parameter.
  abc_to_dq1 : Subsystem
  Freq : Outport
  Vd : Outport  Port=2
  Vq : Outport  Port=3
  Sin_Cos : Outport  Port=4
  wires:
  abc_to_dq1/1(vd) -> Vd/1
  2nd-Order Filter/1(Out) -> Freq/1, Variable Frequency Mean value/1(Freq)
  Variable Frequency Mean value/1(Mean) -> Discrete PI Controller/1(Error)
  Vab_bc (pu)/1 -> abc_to_dq1/1(Vab_bc)
  abc_to_dq1/2(vq) -> Vq/1, Variable Frequency Mean value/2(In)  "Vq"
  Constant4/1 -> Math Function/2
  Integrator/1 -> Math Function/1
  Math Function/1 -> Trigonometric Function/1, Trigonometric Function2/1
  Trigonometric Function/1 -> Mux2/1
  Trigonometric Function2/1 -> Mux2/2
  Mux2/1 -> abc_to_dq1/2(sin_cos), Sin_Cos/1
  Discrete PI Controller/1(Out) -> Integrator/1, Gain10/1  "W"
  Gain10/1 -> Rate Limiter/1
  Rate Limiter/1 -> 2nd-Order Filter/1(In)

== system powerlib_models/Continuous/Dynamic_Load/Break  Alg. Loop ==
  In : Inport  Orientation=left  Port=1  LatchInput=off
  Complex to Real-Imag : ComplexToRealImag  Orientation=left
  Real-Imag to Complex : RealImagToComplex  Orientation=left
  imag : Subsystem  Orientation=left  AncestorBlock=|  mask(Transfer Function with Initial Outputs){N=[1], D=[100e-6  1], Y0=imag(I1_init*exp(-j*Pha_V0*pi/180)), U0=imag(I1_init*exp(-j*Pha_V0*pi/180))}
      | simulink_extras/Additional
      | Linear/Transfer Fcn
      | (with initial outputs)
      mask prompts: N "Numerator:"; D "Denominator:"; Y0 "Initial output:"; U0 "Initial input:"
      mask help: Vector expressions for numerator, and denominator. Coefficients are in descending powers of s.
      mask init:
      | [A,B,C,Dd]=tf2ss(N,D);if (isempty(Y0));[m,n]=size(A);X0=zeros(1,m); end; if (isempty(U0));[m,p]=size(B);U0=zeros(1,p);end;X0=getxo(A,B,C,Dd,U0,Y0,0);
      mask Help: Specify the initial output for the transfer function.  An optimization routine attempts to determine the appropriate initial states so that the specified initial output is achieved.  For more details, see the m-file getxo.m
      mask Display: dpoly(N,D,'s')
  real : Subsystem  Orientation=left  AncestorBlock=|  mask(Transfer Function with Initial Outputs){N=[1], D=[100e-6  1], Y0=real(I1_init*exp(-j*Pha_V0*pi/180)), U0=real(I1_init*exp(-j*Pha_V0*pi/180))}
      | simulink_extras/Additional
      | Linear/Transfer Fcn
      | (with initial outputs)
      mask prompts: N "Numerator:"; D "Denominator:"; Y0 "Initial output:"; U0 "Initial input:"
      mask help: Vector expressions for numerator, and denominator. Coefficients are in descending powers of s.
      mask init:
      | [A,B,C,Dd]=tf2ss(N,D);if (isempty(Y0));[m,n]=size(A);X0=zeros(1,m); end; if (isempty(U0));[m,p]=size(B);U0=zeros(1,p);end;X0=getxo(A,B,C,Dd,U0,Y0,0);
      mask Help: Specify the initial output for the transfer function.  An optimization routine attempts to determine the appropriate initial states so that the specified initial output is achieved.  For more details, see the m-file getxo.m
      mask Display: dpoly(N,D,'s')
  Out : Outport  Orientation=left
  wires:
  In/1 -> Complex to Real-Imag/1
  Real-Imag to Complex/1 -> Out/1
  Complex to Real-Imag/1 -> real/1(In1)
  real/1(Out1) -> Real-Imag to Complex/1
  Complex to Real-Imag/2 -> imag/1(In1)
  imag/1(Out1) -> Real-Imag to Complex/2

== system powerlib_models/Continuous/Dynamic_Load/Positive Sequence  current ==
  note: I1= (S/V1)'
  note: V>Vmin :
      |
      |    P=Po*(V/Vo)^np
      |    Q=Qo*(V/Vo)^np
  note: V<Vmin
      | Constant impedance load :
      |
      |  P=Po*kp*V^2
      | Q=Qo*kq*V^2
  note: kp=Vmin^(np-2)/Vo^np
      | kq=Vmin^(nq-2)/Vo^nq
  V1(pu) : Inport  Port=1  LatchInput=off
  S_ext : Inport  Port=2  LatchInput=off
  Complex to Magnitude-Angle : ComplexToMagnitudeAngle  Output=Magnitude
  Complex to Real-Imag1 : ComplexToRealImag
  Conj1 : Math  Operator=conj  SaturateOnIntegerOverflow=on
  Math Function : Math  Operator=square  SaturateOnIntegerOverflow=on
  Mux1 : Mux  Inputs=3
  Mux2 : Mux  Inputs=2
  Mux3 : Mux  Inputs=2
  P0/ (Vo^np) : Gain  Gain=P0/(Mag_V0^np)  SaturateOnIntegerOverflow=on
  PQ_ext : Constant  Value=PQext
  Product : Product  Inputs=/*  SaturateOnIntegerOverflow=on  InputSameDT=on
  Q0/(Vo^nq) : Gain  Gain=Q0/(Mag_V0^nq)  SaturateOnIntegerOverflow=on
  Real-Imag to Complex : RealImagToComplex
  Switch1 : Switch  Threshold=0.5  InputSameDT=on
  Switch3 : Switch  Threshold=Vmin  InputSameDT=on
  Switch4 : Switch  Threshold=Vmin  InputSameDT=on
  TF_P : Subsystem  mask(Transfer function){T1=Tp1, T2=Tp2, V_Init=P0}
      mask prompts: T1 "Time constant T1 (s):"; T2 "Time constant T2 (s):"; V_Init "Initial input and output :"
      mask help:
      | This block implements a continuous transfer function:
      |
      |          1+T1s
      | H(s)= ------
      |          1+T2s
      |
      | States are initialized according to  initial input and output value so that simulation starts in steady state.
      mask init:
      | numc=[T1 1];
      | denc=[T2 1];
      | [Ac,Bc,Cc,Dc]=tf2ss(numc,denc);
      | 
      | % Compute Initial states
      | I=eye(size(Ac));
      | x0c=inv(-Ac)*Bc*V_Init;
      mask Display: disp('1+T1s\n---\n1+T2s')
  TF_Q : Subsystem  mask(Transfer function){T1=Tq1, T2=Tq2, V_Init=Q0}
      mask prompts: T1 "Time constant T1 (s):"; T2 "Time constant T2 (s):"; V_Init "Initial input and output :"
      mask help:
      | This block implements a continuous transfer function:
      |
      |          1+T1s
      | H(s)= ------
      |          1+T2s
      |
      | States are initialized according to  initial input and output value so that simulation starts in steady state.
      mask init:
      | numc=[T1 1];
      | denc=[T2 1];
      | [Ac,Bc,Cc,Dc]=tf2ss(numc,denc);
      | 
      | % Compute Initial states
      | I=eye(size(Ac));
      | x0c=inv(-Ac)*Bc*V_Init;
      mask Display: disp('1+T1s\n---\n1+T2s')
  V^nq : Fcn  Expr=u[1]^u[2]
  V^nq , : Fcn  Expr=u[1]^u[2]
  Vmin^(np-2) : Gain  Gain=Vmin^(np-2)  SaturateOnIntegerOverflow=on
  Vmin^(nq-2) : Gain  Gain=Vmin^(nq-2)  SaturateOnIntegerOverflow=on
  np : Constant  Value=np
  nq : Constant  Value=nq
  pu>V : Gain  Gain=Vnom*sqrt(3)/sqrt(2)  SaturateOnIntegerOverflow=on
  I1(A) : Outport
  VPQ : Outport  Port=2
  wires:
  TF_Q/1(Out1) -> Real-Imag to Complex/2
  TF_P/1(Out1) -> Real-Imag to Complex/1
  Complex to Real-Imag1/2 -> Mux1/3
  Complex to Real-Imag1/1 -> Mux1/2
  Mux1/1 -> VPQ/1
  Complex to Magnitude-Angle/1 -> Mux1/1, Switch4/2, Switch3/2, Mux2/1, Mux3/1, Math Function/1
  pu>V/1 -> Product/1
  PQ_ext/1 -> Switch1/2
  S_ext/1 -> Switch1/1
  Real-Imag to Complex/1 -> Switch1/3  "S_dyn"
  Switch1/1 -> Complex to Real-Imag1/1, Product/2  "S=P+jQ"
  Conj1/1 -> I1(A)/1
  Product/1 -> Conj1/1
  Switch4/1 -> Q0/(Vo^nq)/1
  P0/ (Vo^np)/1 -> TF_P/1(In1)
  Q0/(Vo^nq)/1 -> TF_Q/1(In1)
  Switch3/1 -> P0/ (Vo^np)/1
  np/1 -> Mux2/2
  Mux2/1 -> V^nq ,/1
  nq/1 -> Mux3/2
  Mux3/1 -> V^nq/1
  V1(pu)/1 -> pu>V/1, Complex to Magnitude-Angle/1
  V^nq/1 -> Switch4/1
  Math Function/1 -> Vmin^(np-2)/1, Vmin^(nq-2)/1
  Vmin^(np-2)/1 -> Switch3/3
  V^nq ,/1 -> Switch3/1
  Vmin^(nq-2)/1 -> Switch4/3

== system powerlib_models/Continuous/Dynamic_Load/Variable Frequency Mean value1 ==
  note: Pierre Giroux, Gilbert Sybille
      | Power System Simulation Laboratory
      | IREQ, Hydro-Quebc
  note: Mean Value (Variable frequency)
  Freq : Inport  Port=1  LatchInput=off
  In : Inport  Port=2  LatchInput=off
  Constant : Constant  Value=Vinit
  Integrator : Integrator
  Number of samples per cycle : Fcn  Expr=1/u[1]
  Product : Product  SaturateOnIntegerOverflow=on  InputSameDT=on
  Step : Step  Time=1/Finit  SampleTime=0
  Sum7 : Sum  Inputs=-+  SaturateOnIntegerOverflow=on  InputSameDT=on
  Switch : Switch  Threshold=0.5  InputSameDT=on
  To avoid division by zero : Saturate  Orientation=down  UpperLimit=1e6  LowerLimit=1e-6
  Variable Transport Delay : VariableTransportDelay  MaximumDelay=1/40  MaximumPoints=4096
  Mean : Outport
  wires:
  In/1 -> Integrator/1  "In"
  Product/1 -> Switch/1  "Mean value"
  Variable Transport Delay/1 -> Sum7/1
  Sum7/1 -> Product/1
  Integrator/1 -> Sum7/2, Variable Transport Delay/1
  Freq/1 -> Product/2, To avoid division by zero/1  "Freq"
  Constant/1 -> Switch/3
  Switch/1 -> Mean/1
  To avoid division by zero/1 -> Number of samples per cycle/1  "Freq"
  Step/1 -> Switch/2
  Number of samples per cycle/1 -> Variable Transport Delay/2  "Delay"

== system powerlib_models/Continuous/Dynamic_Load/Variable Frequency Mean value2 ==
  note: Mean Value (Variable frequency)
  note: Pierre Giroux, Gilbert Sybille
      | Power System Simulation Laboratory
      | IREQ, Hydro-Quebc
  Freq : Inport  Port=1  LatchInput=off
  In : Inport  Port=2  LatchInput=off
  Constant : Constant  Value=Vinit
  Integrator : Integrator
  Number of samples per cycle : Fcn  Expr=1/u[1]
  Product : Product  SaturateOnIntegerOverflow=on  InputSameDT=on
  Step : Step  Time=1/Finit  SampleTime=0
  Sum7 : Sum  Inputs=-+  SaturateOnIntegerOverflow=on  InputSameDT=on
  Switch : Switch  Threshold=0.5  InputSameDT=on
  To avoid division by zero : Saturate  Orientation=down  UpperLimit=1e6  LowerLimit=1e-6
  Variable Transport Delay : VariableTransportDelay  MaximumDelay=1/40  MaximumPoints=4096
  Mean : Outport
  wires:
  Number of samples per cycle/1 -> Variable Transport Delay/2  "Delay"
  Step/1 -> Switch/2
  To avoid division by zero/1 -> Number of samples per cycle/1  "Freq"
  Switch/1 -> Mean/1
  Constant/1 -> Switch/3
  Freq/1 -> To avoid division by zero/1, Product/2  "Freq"
  Integrator/1 -> Variable Transport Delay/1, Sum7/2
  Sum7/1 -> Product/1
  Variable Transport Delay/1 -> Sum7/1
  Product/1 -> Switch/1  "Mean value"
  In/1 -> Integrator/1  "In"

== system powerlib_models/Continuous/Excitation_System/Damping kf.s | (tf.s+1) ==
  In1 : Inport  Port=1  LatchInput=off
  State Space : StateSpace  A=A  B=B  C=C  D=Dd  X0=X0
  Out1 : Outport  InitialOutput=0
  wires:
  In1/1 -> State Space/1
  State Space/1 -> Out1/1

== system powerlib_models/Continuous/Excitation_System/Exciter 1| (te.s+ke) ==
  In1 : Inport  Port=1  LatchInput=off
  State Space : StateSpace  A=A  B=B  C=C  D=Dd  X0=X0
  Out1 : Outport  InitialOutput=0
  wires:
  In1/1 -> State Space/1
  State Space/1 -> Out1/1

== system powerlib_models/Continuous/Excitation_System/Lead Lag Compensator (tc.s+1) | (tb.s+1) ==
  In1 : Inport  Port=1  LatchInput=off
  State Space : StateSpace  A=A  B=B  C=C  D=Dd  X0=X0
  Out1 : Outport  InitialOutput=0
  wires:
  In1/1 -> State Space/1
  State Space/1 -> Out1/1

== system powerlib_models/Continuous/Excitation_System/Low Pass Filter 1 | (tr.s+1) ==
  In1 : Inport  Port=1  LatchInput=off
  State Space : StateSpace  A=A  B=B  C=C  D=Dd  X0=X0
  Out1 : Outport  InitialOutput=0
  wires:
  In1/1 -> State Space/1
  State Space/1 -> Out1/1

== system powerlib_models/Continuous/Excitation_System/Main Regulator ka | (ta.s +1) ==
  In1 : Inport  Port=1  LatchInput=off
  State Space : StateSpace  A=A  B=B  C=C  D=Dd  X0=X0
  Out1 : Outport  InitialOutput=0
  wires:
  In1/1 -> State Space/1
  State Space/1 -> Out1/1

== system powerlib_models/Continuous/Excitation_System/Proportionnal Saturation ==
  Efd : Inport  Port=1  LatchInput=off
  Vtf : Inport  Port=2  LatchInput=off
  Constant : Constant  Value=kp
  Constant1 : Constant  Value=efmin
  Constant3 : Constant  Value=0
  Data Type  Conversion{,1..3} (4 alike) : DataTypeConversion  OutDataTypeMode=double  SaturateOnIntegerOverflow=on  RndMeth=Zero
  Logical Operator : Logic
  Logical Operator1 : Logic  Operator=NOT  Inputs=1
  Logical Operator2 : Logic  Operator=NOT  Inputs=1
  Product : Product  SaturateOnIntegerOverflow=on  InputSameDT=on
  Product1 : Product  SaturateOnIntegerOverflow=on  InputSameDT=on
  Product2 : Product  SaturateOnIntegerOverflow=on  InputSameDT=on
  Relational Operator : RelationalOperator  Operator===  InputSameDT=on
  Relational Operator1 : RelationalOperator  Operator=<  InputSameDT=on
  Relational Operator2 : RelationalOperator  Operator=>  InputSameDT=on
  Sum : Sum  SaturateOnIntegerOverflow=on  InputSameDT=on
  Sum1 : Sum  Inputs=+++  SaturateOnIntegerOverflow=on  InputSameDT=on
  Vfdmax : Gain  Gain=efmax  SaturateOnIntegerOverflow=on
  Vfdmax1 : Gain  Gain=kp  SaturateOnIntegerOverflow=on
  Ef : Outport  InitialOutput=0
  wires:
  Data Type  Conversion3/1 -> Vfdmax/1
  Relational Operator/1 -> Data Type  Conversion3/1
  Data Type  Conversion2/1 -> Product2/1
  Logical Operator2/1 -> Data Type  Conversion2/1
  Data Type  Conversion1/1 -> Product1/2
  Logical Operator1/1 -> Data Type  Conversion1/1
  Data Type  Conversion/1 -> Product/2
  Logical Operator/1 -> Data Type  Conversion/1
  Product1/1 -> Sum1/2
  Product2/1 -> Sum1/3
  Product/1 -> Sum1/1
  Sum1/1 -> Ef/1
  Efd/1 -> Product/1, Relational Operator1/1, Relational Operator2/1
  Constant1/1 -> Product1/1, Relational Operator2/2
  Relational Operator1/1 -> Logical Operator/2, Logical Operator2/1
  Relational Operator2/1 -> Logical Operator/1, Logical Operator1/1
  Sum/1 -> Relational Operator1/2, Product2/2
  Vfdmax1/1 -> Sum/1
  Vfdmax/1 -> Sum/2
  Constant3/1 -> Relational Operator/2
  Constant/1 -> Relational Operator/1
  Vtf/1 -> Vfdmax1/1

== system powerlib_models/Continuous/GTO-IGBT Bridge/Diode Logic ==
  note: Note : Block D1 (D2) if D2 (D1) is triggered (no Cs)
  Vak : Inport  Port=1  LatchInput=off
  Ipos : Inport  Port=2  LatchInput=off
  G : Inport  Port=3  LatchInput=off
  0 2 : Constant  Value=0
  0 3 : Constant  Value=Cs==inf
  1 : Logic
  2 : Logic  Operator=OR
  3 : Logic  Operator=OR
  Block D : Selector  Orientation=up  Elements=Selec_Diode  InputPortWidth=nb_switch
  Blocking Diodes : Subsystem
  Data Type  Conversion3 : DataTypeConversion  OutDataTypeMode=boolean  SaturateOnIntegerOverflow=on  RndMeth=Zero
  Logical Operator3 : Logic  Operator=NOT
  Trig.  Diodes (No Snubber Capacitance) : Subsystem  TreatAsAtomicUnit=on
  b6 : RelationalOperator  Operator=>  InputSameDT=on
  status : Outport  InitialOutput=0
  wires:
  0 3/1 -> Trig.  Diodes (No Snubber Capacitance)/Enable
  Ipos/1 -> Trig.  Diodes (No Snubber Capacitance)/2(Ipos)
  G/1 -> Trig.  Diodes (No Snubber Capacitance)/1(G), Blocking Diodes/1(G)
  0 2/1 -> b6/2
  Vak/1 -> b6/1
  Blocking Diodes/1(Block.D) -> 3/1
  2/1 -> status/1
  1/1 -> 2/1
  Logical Operator3/1 -> 1/2
  3/1 -> Logical Operator3/1
  Trig.  Diodes (No Snubber Capacitance)/1(Trig D) -> 2/2, Block D/1
  Block D/1 -> 3/2
  b6/1 -> Data Type  Conversion3/1
  Data Type  Conversion3/1 -> 1/1

== system powerlib_models/Continuous/GTO-IGBT Bridge/GTO Logic ==
  Vak : Inport  Port=1  LatchInput=off
  G : Inport  Port=2  LatchInput=off
  " " : RelationalOperator  Operator=>  InputSameDT=on
  "    " : Constant  Value=0
  ". " : Logic
  Data Type  Conversion1 : DataTypeConversion  OutDataTypeMode=boolean  SaturateOnIntegerOverflow=on  RndMeth=Zero
  Data Type  Conversion3 : DataTypeConversion  OutDataTypeMode=boolean  SaturateOnIntegerOverflow=on  RndMeth=Zero
  Data Type  Conversion4 : DataTypeConversion  OutDataTypeMode=boolean  SaturateOnIntegerOverflow=on  RndMeth=Zero
  Vpos : Constant  Value=0
  b : RelationalOperator  Operator=>  InputSameDT=on
  status : Outport  InitialOutput=0
  wires:
  ". "/1 -> status/1
  Vak/1 -> b/1
  Vpos/1 -> b/2
  G/1 -> " "/1
  b/1 -> Data Type  Conversion1/1
  Data Type  Conversion1/1 -> ". "/1
  " "/1 -> Data Type  Conversion3/1
  Data Type  Conversion3/1 -> ". "/2
  "    "/1 -> Data Type  Conversion4/1
  Data Type  Conversion4/1 -> " "/2

== system powerlib_models/Continuous/GTO-IGBT Bridge/Tail  ==
  Iak : Inport  Port=1  LatchInput=off
  switch : Inport  Port=2  LatchInput=off
  Enable : EnablePort  StatesWhenEnabling=reset
  1 : Constant
  2 : Constant  Value=(Tf+Tt)>0  OutDataTypeMode=double
  Integrator : Integrator  ExternalReset=falling
  Look-Up Table : Lookup  DialogController=Simulink.DDGSource  InputValues="[  0   Tf+eps Tf+Tt+2*eps  Tf+Tt+3*eps]"  OutputValues="[  1   0.1*(Tt>0) 0 0]"  SaturateOnIntegerOverflow=on
  Memory : Memory  Orientation=left  InheritSampleTime=on
  Product : Product  Inputs=3  SaturateOnIntegerOverflow=on  InputSameDT=on
  Switch : Switch  Threshold=0.5  InputSameDT=on
  itail : Outport  InitialOutput=0
  wires:
  2/1 -> Product/3
  Look-Up Table/1 -> Product/1
  1/1 -> Integrator/1
  Iak/1 -> Switch/1
  switch/1 -> Switch/2, Integrator/2
  Integrator/1 -> Look-Up Table/1
  Product/1 -> itail/1
  Switch/1 -> Product/2, Memory/1
  Memory/1 -> Switch/3
